simulink model "AcermanDynExt"  (R2021a)
settings: Solver=FixedStepAuto  StartTime=0.0  StopTime=simTime  RelTol=1e-3
values from neighbouring files (symbols this model uses):
  a = 2    [Ackerman_init.m]
  a0 = 1    [Ackerman_init.m]
  a1 = 4    [Ackerman_init.m]
  a2 = 3    [Ackerman_init.m]
  b = 1.05*a    (= 2.1)    [Ackerman_init.m]
  Change = 0    [Ackerman_init.m]
  k0 = 1    [Ackerman_init.m]
  k1 = place(Ad,bd,pd)    [Ackerman_init.m]
  k2 = place(Ac,bc,lambdatr')    [Ackerman_init.m]
  l = ylabel('$\omega(t)$' )    [Ackerman_init.m]
  pathType = 1    [Ackerman_init.m]
  phi0 = 0    [Ackerman_init.m]
  r = 2    [Ackerman_init.m]
  ref0 = [0 0]'    [Ackerman_init.m]
  refType = 1    [Ackerman_init.m]
  T = 0.1    [Ackerman_init.m]
  theta0 = pi/2    (= 1.57079632679)    [Ackerman_init.m]
  v0 = 1    [Ackerman_init.m]
  v_ref = 2    [Ackerman_init.m]
  x0 = 1    [Ackerman_init.m]
  y0 = 1    [Ackerman_init.m]
libraries: robotmobilelib x5
(part 4 of 4)

== matlab function AcermanDynExt/MATLAB Function ==
  data: v input; a input; u input; v output; a output; T parameter
function [v,a] = fcn(v,a, u, T)

A = [1 T;0 1];
B = [T^2/2 ; T];

states = A*[v;a] + B*u;
v = states(1);
a = states(2);

== matlab function AcermanDynExt/MATLAB Function14 ==
  data: u1 input; y output; u2 input; x0 parameter; y0 parameter
function y = fcn(u1, u2, x0, y0)

if x0 == 1 && y0 == 1
    y = u2;
else
    y = u1;
end

== matlab function AcermanDynExt/MATLAB Function13 ==
  data: x output; state input; y output; theta output; emr output; pathType parameter; r parameter; a parameter; b parameter
function [x, y, theta, emr] = fcn(state, pathType, r, a, b)

x = state(1);
y = state(2);
theta = state(3);
if pathType == 1
    emr = x^2+y^2 - r^2;
else
    emr = (x^2+y^2+a^2)^2-4*a^2*x^2-b^4;
    
end

== matlab function AcermanDynExt/MATLAB Function5 ==
  data: state input; vold input; vd input; v_ref input; pathType parameter; k0 parameter; r parameter; l parameter; utn output; utr output; Change parameter; k2 parameter
function [utn,utr] = MATLAB_Function5(state, vold, vd, v_ref, pathType, k0, r, l, Change, k2)

x = state(1); y = state(2); theta = state(3); phi = state(4);
eta1 = vold; eta2 = vd;

if pathType == 1
    D = [ -(y*cos(theta) - x*sin(theta))/(x^2 + y^2), (eta1^2*(x*cos(theta) + y*sin(theta)))/(l*cos(phi)^2*(x^2 + y^2));
            2*x*cos(theta) + 2*y*sin(theta),           (2*eta1^2*(y*cos(theta) - x*sin(theta)))/(l*cos(phi)^2)];
    F  = [  (eta1*(sin(phi)*x^2 - 2*l*cos(phi)*sin(theta)*x + sin(phi)*y^2 + 2*l*cos(phi)*cos(theta)*y)*(eta1^2*l*x^2*cos(phi) - 3*eta1^2*l*y^2*cos(phi) + eta1^2*y^3*cos(theta)*sin(phi) - eta1^2*x^3*sin(phi)*sin(theta) + eta1^2*x^2*y*cos(theta)*sin(phi) - eta1^2*x*y^2*sin(phi)*sin(theta) - 4*eta1^2*l*x^2*cos(phi)*cos(theta)^2 + 4*eta1^2*l*y^2*cos(phi)*cos(theta)^2 + 3*eta2*l*x^3*cos(phi)*cos(theta) + 3*eta2*l*y^3*cos(phi)*sin(theta) + 3*eta2*l*x*y^2*cos(phi)*cos(theta) + 3*eta2*l*x^2*y*cos(phi)*sin(theta) - 8*eta1^2*l*x*y*cos(phi)*cos(theta)*sin(theta)))/(l^2*cos(phi)^2*(x^2 + y^2)^3);
                                                                                                                                                                                                                                                                                                                                           (2*eta1*(3*eta2*l^2*cos(phi)^2*sin(theta)^2 - eta1^2*x*cos(theta)*sin(phi)^2 - eta1^2*y*sin(phi)^2*sin(theta) + 3*eta2*l^2*cos(phi)^2*cos(theta)^2 + 3*eta2*l*y*cos(phi)*cos(theta)*sin(phi) - 3*eta2*l*x*cos(phi)*sin(phi)*sin(theta)))/(l^2*cos(phi)^2)];
else

    D = [ -(y*cos(theta)-x*sin(theta))/(x^2 + y^2),  (eta1^2*(x*cos(theta)+y*sin(theta)))/(cos(phi)^2*(x^2+y^2));
         4*x*cos(theta)*(x^2 + y^2-9)+4*y*sin(theta)*(x^2 + y^2+9),    eta1*(tan(phi)^2+1)*(4*y*eta1*cos(theta)*(x^2 + y^2+9)-4*x*eta1*sin(theta)*(x^2 + y^2-9))];
 
     F  = [ (eta1*(sin(phi)*x^2-2*cos(phi)*sin(theta)*x+sin(phi)*y^2+2*cos(theta)*cos(phi)*y)*(x^2*eta1^2*cos(phi)-3*y^2*eta1^2*cos(phi)-4*x^2*eta1^2*cos(theta)^2*cos(phi)+4*y^2*eta1^2*cos(theta)^2*cos(phi)+3*x^3*eta2*cos(theta)*cos(phi)+3*y^3*eta2*cos(phi)*sin(theta)+y^3*eta1^2*cos(theta)*sin(phi)-x^3*eta1^2*sin(theta)*sin(phi)+x^2*y*eta1^2*cos(theta)*sin(phi)-x*y^2*eta1^2*sin(theta)*sin(phi)+3*x*y^2*eta2*cos(theta)*cos(phi)+3*x^2*y*eta2*cos(phi)*sin(theta)-8*x*y*eta1^2*cos(theta)*cos(phi)*sin(theta)))/(cos(phi)^2*(x^2 + y^2)^3);
       (36*x*eta1^3*cos(theta) + 108*eta1*eta2*cos(phi)^2 - 36*y*eta1^3*sin(theta) - 4*x^3*eta1^3*cos(theta) - 4*y^3*eta1^3*sin(theta) + 4*x^3*eta1^3*cos(theta)*cos(phi)^2 + 4*y^3*eta1^3*cos(phi)^2*sin(theta) - 4*x*y^2*eta1^3*cos(theta) + 12*x^2*eta1*eta2*cos(phi)^2 + 36*y^2*eta1*eta2*cos(phi)^2 - 12*x*y*eta1^3*sin(2*phi) - 4*x^2*y*eta1^3*sin(theta) - 12*x*eta1^3*cos(theta)*cos(phi)^2 - 216*eta1*eta2*cos(theta)^2*cos(phi)^2 + 60*y*eta1^3*cos(phi)^2*sin(theta) + 4*x*y^2*eta1^3*cos(theta)*cos(phi)^2 + 24*x^2*eta1*eta2*cos(theta)^2*cos(phi)^2 - 24*y^2*eta1*eta2*cos(theta)^2*cos(phi)^2 + 4*x^2*y*eta1^3*cos(phi)^2*sin(theta) + 216*eta1^3*cos(theta)*cos(phi)*sin(theta)*sin(phi) + 48*x*y*eta1^3*cos(theta)^2*cos(phi)*sin(phi) + 108*y*eta1*eta2*cos(theta)*cos(phi)*sin(phi) + 108*x*eta1*eta2*cos(phi)*sin(theta)*sin(phi) - 24*x^2*eta1^3*cos(theta)*cos(phi)*sin(theta)*sin(phi) + 24*y^2*eta1^3*cos(theta)*cos(phi)*sin(theta)*sin(phi) + 12*y^3*eta1*eta2*cos(theta)*cos(phi)*sin(phi) - 12*x^3*eta1*eta2*cos(phi)*sin(theta)*sin(phi) + 48*x*y*eta1*eta2*cos(theta)*cos(phi)^2*sin(theta) + 12*x^2*y*eta1*eta2*cos(theta)*cos(phi)*sin(phi) - 12*x*y^2*eta1*eta2*cos(phi)*sin(theta)*sin(phi))/cos(phi)^2];
    
end

  
Di = pinv(D);

if pathType == 1
    alpha = x^2+y^2 - r^2;
    psi1 = x^2+y^2-r^2; %
    psi2 = 2*eta1*(x*cos(theta) + y*sin(theta));
    psi3 = 2*eta1^2*cos(theta)^2 + 2*eta1^2*sin(theta)^2 + eta2*(2*x*cos(theta) + 2*y*sin(theta)) + (2*eta1^2*tan(phi)*(y*cos(theta) - x*sin(theta)))/l;

else
    a       = 3; b       = 1.05*a;
    alpha = (x^2+y^2+a^2)^2-4*a^2*x^2-b^4; % defines the path
    psi1 = (x^2+y^2+a^2)^2-4*a^2*x^2-b^4;
    psi2 = 4*x*eta1*cos(theta)*(x^2 + y^2 - 9) + 4*y*eta1*sin(theta)*(x^2 + y^2 + 9);
    psi3 = eta2*(4*x*cos(theta)*(x^2 + y^2 - 9) + 4*y*sin(theta)*(x^2 + y^2 + 9)) + eta1*cos(theta)*(8*x^2*eta1*cos(theta) + 4*eta1*cos(theta)*(x^2 + y^2 - 9) + 8*x*y*eta1*sin(theta)) + eta1*sin(theta)*(8*y^2*eta1*sin(theta) + 4*eta1*sin(theta)*(x^2 + y^2 + 9) + 8*x*y*eta1*cos(theta)) + eta1*tan(phi)*(4*y*eta1*cos(theta)*(x^2 + y^2 + 9) - 4*x*eta1*sin(theta)*(x^2 + y^2 - 9));
end


if alpha < 1e-2 && Change == 1
    ref = 2*v_ref;
else
    ref = v_ref;
end

v1 = -k0*(eta1-ref)-k0*eta2; 
v2 = k2*[psi1;psi2;psi3];
u  = Di*([v1;v2]-F);
utn = u(1); 
utr = u(2);

== matlab function AcermanDynExt/MATLAB Function1 ==
  data: x output; state input; y output; theta output; emr output; pathType parameter; r parameter; a parameter; b parameter
function [x, y, theta, emr] = fcn(state, pathType, r, a, b)

x = state(1);
y = state(2);
theta = state(3);
if pathType == 1
    emr = x^2+y^2 - r^2;
else
    emr = (x^2+y^2+a^2)^2-4*a^2*x^2-b^4;
    
end

== matlab function AcermanDynExt/MATLAB Function2 ==
  data: state input; ve input; ved input; v_ref input; pathType parameter; k0 parameter; r parameter; l parameter; utn output; utr output; Change parameter; k2 parameter
function [utn,utr] = MATLAB_Function2(state, ve, ved,v_ref, pathType, k0, r, l, Change, k2)

x = state(1); y = state(2); theta = state(3); phi = state(4);
eta1 = ve; eta2 = ved;


if pathType == 1
    D = [ -(y*cos(theta) - x*sin(theta))/(x^2 + y^2), (eta1^2*(x*cos(theta) + y*sin(theta)))/(l*cos(phi)^2*(x^2 + y^2));
            2*x*cos(theta) + 2*y*sin(theta),           (2*eta1^2*(y*cos(theta) - x*sin(theta)))/(l*cos(phi)^2)];
    F  = [  (eta1*(sin(phi)*x^2 - 2*l*cos(phi)*sin(theta)*x + sin(phi)*y^2 + 2*l*cos(phi)*cos(theta)*y)*(eta1^2*l*x^2*cos(phi) - 3*eta1^2*l*y^2*cos(phi) + eta1^2*y^3*cos(theta)*sin(phi) - eta1^2*x^3*sin(phi)*sin(theta) + eta1^2*x^2*y*cos(theta)*sin(phi) - eta1^2*x*y^2*sin(phi)*sin(theta) - 4*eta1^2*l*x^2*cos(phi)*cos(theta)^2 + 4*eta1^2*l*y^2*cos(phi)*cos(theta)^2 + 3*eta2*l*x^3*cos(phi)*cos(theta) + 3*eta2*l*y^3*cos(phi)*sin(theta) + 3*eta2*l*x*y^2*cos(phi)*cos(theta) + 3*eta2*l*x^2*y*cos(phi)*sin(theta) - 8*eta1^2*l*x*y*cos(phi)*cos(theta)*sin(theta)))/(l^2*cos(phi)^2*(x^2 + y^2)^3);
                                                                                                                                                                                                                                                                                                                                           (2*eta1*(3*eta2*l^2*cos(phi)^2*sin(theta)^2 - eta1^2*x*cos(theta)*sin(phi)^2 - eta1^2*y*sin(phi)^2*sin(theta) + 3*eta2*l^2*cos(phi)^2*cos(theta)^2 + 3*eta2*l*y*cos(phi)*cos(theta)*sin(phi) - 3*eta2*l*x*cos(phi)*sin(phi)*sin(theta)))/(l^2*cos(phi)^2)];
else

    D = [ -(y*cos(theta)-x*sin(theta))/(x^2 + y^2),  (eta1^2*(x*cos(theta)+y*sin(theta)))/(cos(phi)^2*(x^2+y^2));
         4*x*cos(theta)*(x^2 + y^2-9)+4*y*sin(theta)*(x^2 + y^2+9),    eta1*(tan(phi)^2+1)*(4*y*eta1*cos(theta)*(x^2 + y^2+9)-4*x*eta1*sin(theta)*(x^2 + y^2-9))];
 
     F  = [ (eta1*(sin(phi)*x^2-2*cos(phi)*sin(theta)*x+sin(phi)*y^2+2*cos(theta)*cos(phi)*y)*(x^2*eta1^2*cos(phi)-3*y^2*eta1^2*cos(phi)-4*x^2*eta1^2*cos(theta)^2*cos(phi)+4*y^2*eta1^2*cos(theta)^2*cos(phi)+3*x^3*eta2*cos(theta)*cos(phi)+3*y^3*eta2*cos(phi)*sin(theta)+y^3*eta1^2*cos(theta)*sin(phi)-x^3*eta1^2*sin(theta)*sin(phi)+x^2*y*eta1^2*cos(theta)*sin(phi)-x*y^2*eta1^2*sin(theta)*sin(phi)+3*x*y^2*eta2*cos(theta)*cos(phi)+3*x^2*y*eta2*cos(phi)*sin(theta)-8*x*y*eta1^2*cos(theta)*cos(phi)*sin(theta)))/(cos(phi)^2*(x^2 + y^2)^3);
       (36*x*eta1^3*cos(theta) + 108*eta1*eta2*cos(phi)^2 - 36*y*eta1^3*sin(theta) - 4*x^3*eta1^3*cos(theta) - 4*y^3*eta1^3*sin(theta) + 4*x^3*eta1^3*cos(theta)*cos(phi)^2 + 4*y^3*eta1^3*cos(phi)^2*sin(theta) - 4*x*y^2*eta1^3*cos(theta) + 12*x^2*eta1*eta2*cos(phi)^2 + 36*y^2*eta1*eta2*cos(phi)^2 - 12*x*y*eta1^3*sin(2*phi) - 4*x^2*y*eta1^3*sin(theta) - 12*x*eta1^3*cos(theta)*cos(phi)^2 - 216*eta1*eta2*cos(theta)^2*cos(phi)^2 + 60*y*eta1^3*cos(phi)^2*sin(theta) + 4*x*y^2*eta1^3*cos(theta)*cos(phi)^2 + 24*x^2*eta1*eta2*cos(theta)^2*cos(phi)^2 - 24*y^2*eta1*eta2*cos(theta)^2*cos(phi)^2 + 4*x^2*y*eta1^3*cos(phi)^2*sin(theta) + 216*eta1^3*cos(theta)*cos(phi)*sin(theta)*sin(phi) + 48*x*y*eta1^3*cos(theta)^2*cos(phi)*sin(phi) + 108*y*eta1*eta2*cos(theta)*cos(phi)*sin(phi) + 108*x*eta1*eta2*cos(phi)*sin(theta)*sin(phi) - 24*x^2*eta1^3*cos(theta)*cos(phi)*sin(theta)*sin(phi) + 24*y^2*eta1^3*cos(theta)*cos(phi)*sin(theta)*sin(phi) + 12*y^3*eta1*eta2*cos(theta)*cos(phi)*sin(phi) - 12*x^3*eta1*eta2*cos(phi)*sin(theta)*sin(phi) + 48*x*y*eta1*eta2*cos(theta)*cos(phi)^2*sin(theta) + 12*x^2*y*eta1*eta2*cos(theta)*cos(phi)*sin(phi) - 12*x*y^2*eta1*eta2*cos(phi)*sin(theta)*sin(phi))/cos(phi)^2];
    
end

  
Di = pinv(D);

if pathType == 1
    alpha = x^2+y^2 - r^2;
    psi1 = x^2+y^2-r^2; %
    psi2 = 2*eta1*(x*cos(theta) + y*sin(theta));
    psi3 = 2*eta1^2*cos(theta)^2 + 2*eta1^2*sin(theta)^2 + eta2*(2*x*cos(theta) + 2*y*sin(theta)) + (2*eta1^2*tan(phi)*(y*cos(theta) - x*sin(theta)))/l;

else
    a       = 3; b       = 1.05*a;
    alpha = (x^2+y^2+a^2)^2-4*a^2*x^2-b^4; % defines the path
    psi1 = (x^2+y^2+a^2)^2-4*a^2*x^2-b^4;
    psi2 = 4*x*eta1*cos(theta)*(x^2 + y^2 - 9) + 4*y*eta1*sin(theta)*(x^2 + y^2 + 9);
    psi3 = eta2*(4*x*cos(theta)*(x^2 + y^2 - 9) + 4*y*sin(theta)*(x^2 + y^2 + 9)) + eta1*cos(theta)*(8*x^2*eta1*cos(theta) + 4*eta1*cos(theta)*(x^2 + y^2 - 9) + 8*x*y*eta1*sin(theta)) + eta1*sin(theta)*(8*y^2*eta1*sin(theta) + 4*eta1*sin(theta)*(x^2 + y^2 + 9) + 8*x*y*eta1*cos(theta)) + eta1*tan(phi)*(4*y*eta1*cos(theta)*(x^2 + y^2 + 9) - 4*x*eta1*sin(theta)*(x^2 + y^2 - 9));
end

if alpha < 1e-2 && Change == 1
    ref = 2*v_ref;
else
    ref = v_ref;
end
v1 = -k0*(eta1-ref)-k0*eta2; 
v2 = k2*[psi1;psi2;psi3];

u  = Di*([v1;v2]-F);
utn = u(1); 
utr = u(2);

== matlab function AcermanDynExt/MATLAB Function3 ==
  data: x output; state input; y output; theta output; emr output; pathType parameter; r parameter; a parameter; b parameter
function [x, y, theta, emr] = fcn(state, pathType, r, a, b)

x = state(1);
y = state(2);
theta = state(3);
if pathType == 1
    emr = x^2+y^2 - r^2;
else
    emr = (x^2+y^2+a^2)^2-4*a^2*x^2-b^4;
    
end
